simulink model "Consat1Payload"  (Simulink 7.9)
settings: Solver=ode45  StartTime=0.0  StopTime=10.0  RelTol=1e-3
values from neighbouring files (symbols this model uses):
  pwmAmplitude = [0:0.5:9]'    [Consat1PayloadScript.m]
  pwmDutyCycle = [0:0.1:100]'    [Consat1PayloadScript.m]
undefined symbols (not defined in the file or in its folder): flybackGainSteps
settings Model: Creator=ahubbell  LastModifiedBy=ahubbell

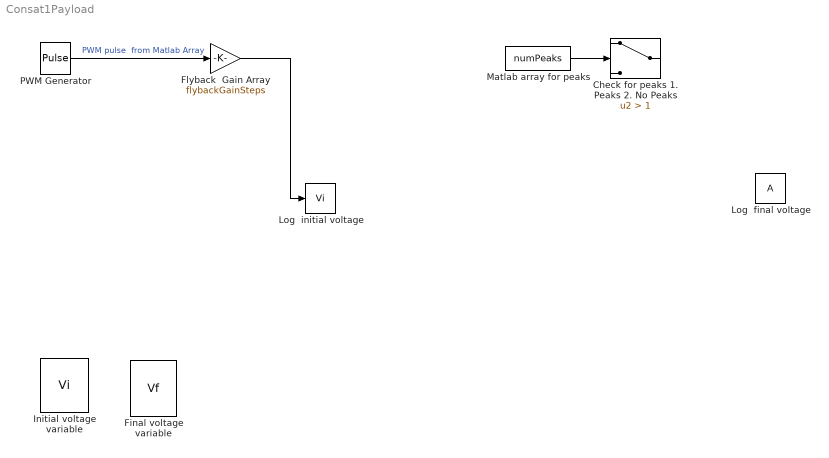
== system Consat1Payload ==
  Check for peaks 1. Peaks 2. No Peaks : Switch  Criteria=u2 > Threshold  Threshold=1
  Final voltage variable : DataStoreMemory  DataStoreName=Vf  ReadBeforeWriteMsg=warning  WriteAfterWriteMsg=warning  WriteAfterReadMsg=warning
  Flyback  Gain Array : Gain  Gain=flybackGainSteps
  Initial voltage variable : DataStoreMemory  DataStoreName=Vi  ReadBeforeWriteMsg=warning  WriteAfterWriteMsg=warning  WriteAfterReadMsg=warning
  Log  final voltage : DataStoreWrite
  Log  initial voltage : DataStoreWrite  DataStoreName=Vi
  Matlab array for peaks : FromWorkspace  VariableName=numPeaks  SampleTime=0
  PWM Generator : DiscretePulseGenerator  PulseType=Time based  Amplitude=pwmAmplitude  Period=10  PulseWidth=pwmDutyCycle
  wires:
  Matlab array for peaks/1 -> Check for peaks 1. Peaks 2. No Peaks/2
  PWM Generator/1 -> Flyback  Gain Array/1  "PWM pulse  from Matlab Array"
  Flyback  Gain Array/1 -> Log  initial voltage/1
